simulink model "Gera_dados_global_LMS"  (Simulink 9.1)
settings: Solver=ode4  StartTime=0.0  StopTime=200  FixedStep=0.005  RelTol=1e-3  EnableMultiTasking=on
settings Model: SuppressorTable=22 serialization::archive 11 0 6 0 0 0 1 0  Creator=Fabricio  LastModifiedBy=marcus
settings DataIOCC: LimitDataPoints=on  SignalLoggingSaveFormat=ModelDataLogs
settings OptimizationCC: ExpressionDepthLimit=2147483647  InitFltsAndDblsToZero=on
settings DebuggingCC: SolverPrmCheckMsg=warning  FcnCallInpInsideContextMsg=warning  StateNameClashWarn=warning
settings GRTTargetCC: GeneratePreprocessorConditionals=Disable all

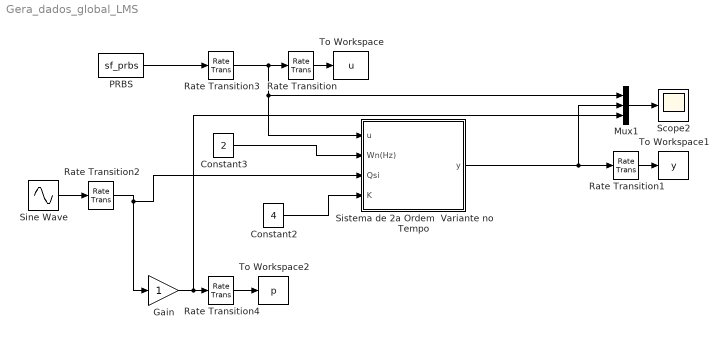
== system Gera_dados_global_LMS ==
  Constant2 : Constant  Value=4
  Constant3 : Constant  Value=2
  Gain : Gain
  Mux1 : Mux  Inputs=3
  PRBS : S-Function  FunctionName=sf_prbs  Parameters=K,N,Ts  SFunctionDeploymentMode=off  EnableBusSupport=off  mask{K=0.1, N=7, Ts=0.12}
      mask prompts: K "Ganho (K):"; N "Número de Células (usar 5, 7 ou 10):"; Ts "Tempo de amostragem (seg):"
      mask Display: disp('P R B S')
  Rate Transition{,1..3} (4 alike) : RateTransition
  Rate Transition4 : RateTransition  InitialCondition=0.05
  Scope2 : Scope
  Sine Wave : Sin  Amplitude=0.4  Bias=0.5  Frequency=0.05  SampleTime=0
  Sistema de 2a Ordem  Variante no Tempo : Subsystem
  To Workspace : ToWorkspace  VariableName=u  SampleTime=0.05
  To Workspace1 : ToWorkspace  VariableName=y  SampleTime=0.05
  To Workspace2 : ToWorkspace  VariableName=p  SampleTime=0.05
  wires:
  Rate Transition/1 -> To Workspace/1
  Rate Transition1/1 -> To Workspace1/1
  Mux1/1 -> Scope2/1
  Rate Transition3/1 -> Rate Transition/1, Sistema de 2a Ordem  Variante no Tempo/1(u), Mux1/1
  Rate Transition4/1 -> To Workspace2/1
  Gain/1 -> Mux1/3, Rate Transition4/1
  Sistema de 2a Ordem  Variante no Tempo/1(y) -> Rate Transition1/1, Mux1/2
  Sine Wave/1 -> Rate Transition2/1
  PRBS/1 -> Rate Transition3/1
  Rate Transition2/1 -> Sistema de 2a Ordem  Variante no Tempo/3(Qsi), Gain/1
  Constant2/1 -> Sistema de 2a Ordem  Variante no Tempo/4(K)
  Constant3/1 -> Sistema de 2a Ordem  Variante no Tempo/2(Wn(Hz))

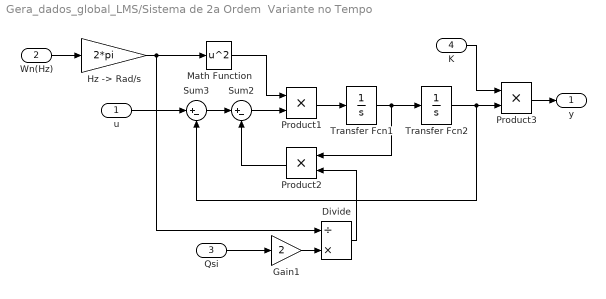
== system Gera_dados_global_LMS/Sistema de 2a Ordem  Variante no Tempo ==
  u : Inport
  Wn(Hz) : Inport  Port=2
  Qsi : Inport  Port=3
  K : Inport  Port=4
  Divide : Product  Inputs=/*
  Gain1 : Gain  Gain=2
  "Hz -> Rad/s" : Gain  Gain=2*pi
  Math Function : Math  Operator=square  SaturateOnIntegerOverflow=on
  Product1 : Product  RndMeth=Zero
  Product2 : Product  RndMeth=Zero
  Product3 : Product  RndMeth=Zero
  Sum2 : Sum  Inputs=|+-
  Sum3 : Sum  Inputs=|+-
  Transfer Fcn1 : TransferFcn  Denominator=[1 0]
  Transfer Fcn2 : TransferFcn  Denominator=[1 0]
  y : Outport
  wires:
  Product1/1 -> Transfer Fcn1/1
  Sum2/1 -> Product1/2
  Product2/1 -> Sum2/2
  Transfer Fcn1/1 -> Product2/1, Transfer Fcn2/1
  Sum3/1 -> Sum2/1
  Transfer Fcn2/1 -> Sum3/2, Product3/2
  Wn(Hz)/1 -> "Hz -> Rad/s"/1
  Math Function/1 -> Product1/1
  Qsi/1 -> Gain1/1
  Gain1/1 -> Divide/2
  Divide/1 -> Product2/2
  u/1 -> Sum3/1
  K/1 -> Product3/1
  Product3/1 -> y/1
  "Hz -> Rad/s"/1 -> Math Function/1, Divide/1
